simulink model "day3"  (R2024a)
settings: Solver=VariableStepAuto  StartTime=0.0  StopTime=10.0  RelTol=1e-3
settings Model: Creator=tusha  LastModifiedBy=tusha

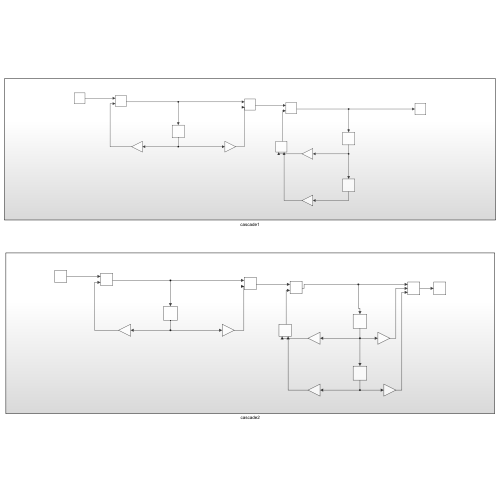
[thumbnail: Simulink's stored preview of the top-level diagram]
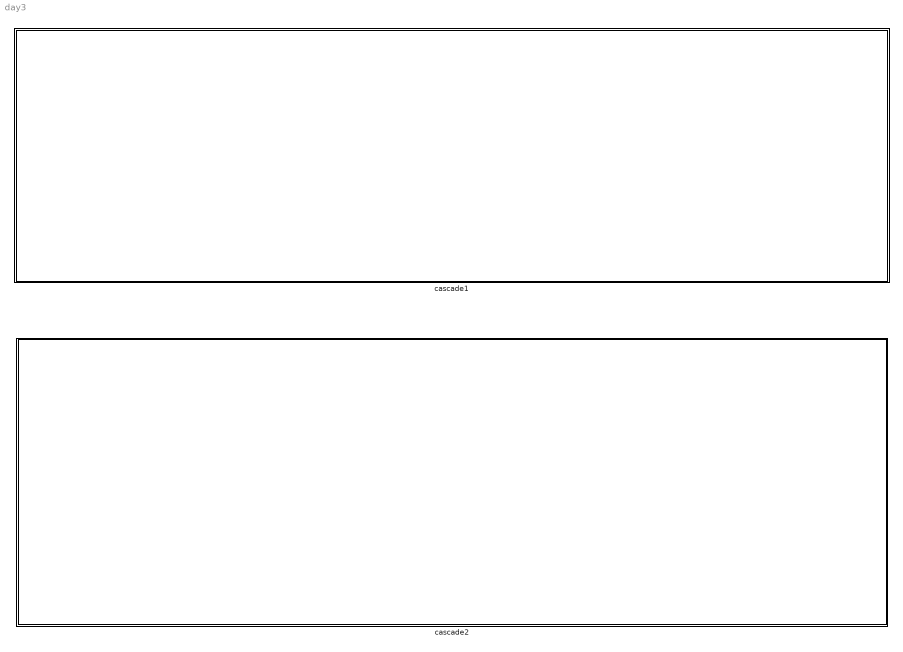
== system day3 ==
  cascade1 : Subsystem
  cascade2 : Subsystem

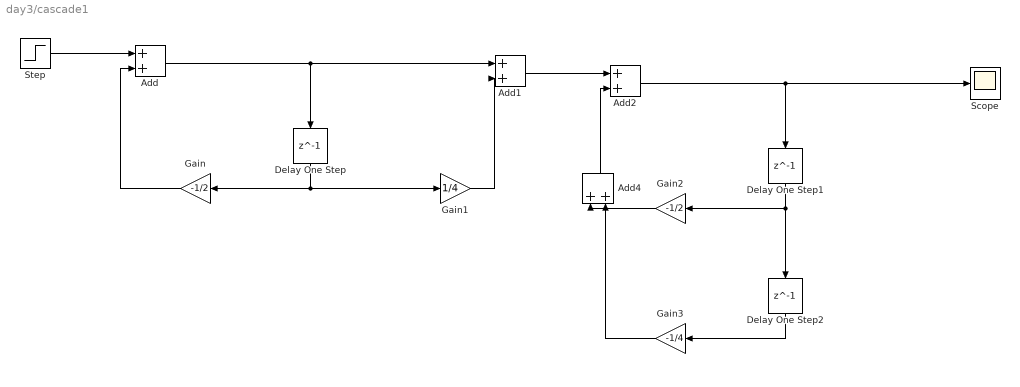
== system day3/cascade1 ==
  Add{,1..2,4} (4 alike) : Sum
  Delay One Step : Delay  DelayLength=1
  Delay One Step1 : Delay  DelayLength=1
  Delay One Step2 : Delay  DelayLength=1
  Gain : Gain  Gain=-1/2
  Gain1 : Gain  Gain=1/4
  Gain2 : Gain  Gain=-1/2
  Gain3 : Gain  Gain=-1/4
  Scope : Scope
  Step : Step  SampleTime=0
  wires:
  Delay One Step/1 -> Gain1/1, Gain/1
  Add/1 -> Add1/1, Delay One Step/1
  Gain1/1 -> Add1/2
  Step/1 -> Add/1
  Gain/1 -> Add/2
  Gain3/1 -> Add4/2
  Delay One Step1/1 -> Delay One Step2/1, Gain2/1
  Add1/1 -> Add2/1
  Add4/1 -> Add2/2
  Add2/1 -> Scope/1, Delay One Step1/1
  Gain2/1 -> Add4/1
  Delay One Step2/1 -> Gain3/1

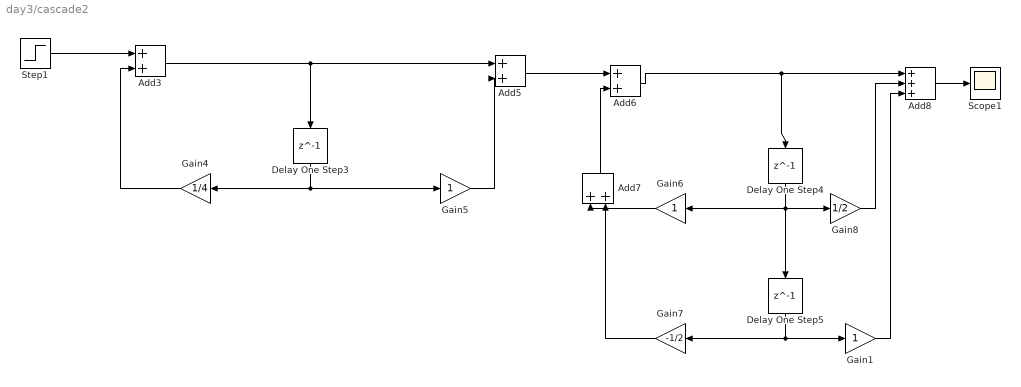
== system day3/cascade2 ==
  Add{3,5..7} (4 alike) : Sum
  Add8 : Sum  Inputs=+++
  Delay One Step3 : Delay  DelayLength=1
  Delay One Step4 : Delay  DelayLength=1
  Delay One Step5 : Delay  DelayLength=1
  Gain1 : Gain
  Gain4 : Gain  Gain=1/4
  Gain5 : Gain
  Gain6 : Gain
  Gain7 : Gain  Gain=-1/2
  Gain8 : Gain  Gain=1/2
  Scope1 : Scope
  Step1 : Step  SampleTime=0
  wires:
  Add5/1 -> Add6/1
  Delay One Step3/1 -> Gain5/1, Gain4/1
  Gain6/1 -> Add7/1
  Gain7/1 -> Add7/2
  Add6/1 -> Delay One Step4/1, Add8/1
  Delay One Step4/1 -> Gain8/1, Delay One Step5/1, Gain6/1
  Add7/1 -> Add6/2
  Add3/1 -> Add5/1, Delay One Step3/1
  Gain5/1 -> Add5/2
  Add8/1 -> Scope1/1
  Gain4/1 -> Add3/2
  Gain8/1 -> Add8/2
  Step1/1 -> Add3/1
  Gain1/1 -> Add8/3
  Delay One Step5/1 -> Gain7/1, Gain1/1
